simulink model "Projet_Final"  (R2024a)
settings: Solver=FixedStepAuto  StartTime=0.0  StopTime=6  FixedStep=Ts  RelTol=1e-3
values from neighbouring files (symbols this model uses):
  A1 = 0.548    [Parameters.m]
  A2 = 116    [Parameters.m]
  A3 = 0.4    [Parameters.m]
  A4 = 5    [Parameters.m]
  A5 = -21    [Parameters.m]
  A6 = 0.0068    [Parameters.m]
  C_Bat = 1e-3    (= 0.001)    [Parameters.m]    (also in Params_Battery_converter.m)
  C_dc = 4.5e-3    (= 0.0045)    [Parameters.m]
  f = 50    [Parameters.m]
  F = 0.0004924    [Parameters.m]
  G = 6.24    [Parameters.m]
  J = J_PMSG    (= 0.2227)    [Parameters.m]
  J_PMSG = 0.2227    [Parameters.m]
  ki_Ibat = 550    [Parameters.m]    (also in Params_Battery_converter.m)
  ki_id_grid = 225    [Parameters.m]
  ki_iq_grid = ki_id_grid    (= 225)    [Parameters.m]
  ki_isd = 13800    [Parameters.m]
  ki_omega = 0.6873    [Parameters.m]
  ki_PLL = 3200    [Parameters.m]
  ki_Q = 0.05    [Parameters.m]
  ki_vdc = C_dc * W_vdc^2    (= 28.8)    [Parameters.m]
  kp_Ibat = 6.28    [Parameters.m]    (also in Params_Battery_converter.m)
  kp_id_grid = 4.5    [Parameters.m]
  kp_iq_grid = kp_id_grid    (= 4.5)    [Parameters.m]
  kp_isd = 2.75    [Parameters.m]
  kp_omega = 3.108    [Parameters.m]
  kp_PLL = 180    [Parameters.m]
  kp_Q = 0.0005    [Parameters.m]
  kp_vdc = 2 * C_dc * W_vdc    (= 0.72)    [Parameters.m]
  Kt = 1.5 * p * Phi_r    (= 0.7164)    [Parameters.m]
  L_Bat = 2e-3    (= 0.002)    [Parameters.m]    (also in Params_Battery_converter.m)
  Lf = 8e-3    (= 0.008)    [Parameters.m]
  Ls = 0.000395    [Parameters.m]
  p = 4    [Parameters.m]
  Phi_r = 0.1194    [Parameters.m]
  R = 3.96    [Parameters.m]
  Rf = 0.01    [Parameters.m]
  rho = 1.225    [Parameters.m]
  Rs = 0.0485    [Parameters.m]
  S = pi*R^2    (= 49.2651993565)    [Parameters.m]
  Ts = 1e-6    (= 1e-06)    [Parameters.m]
  Vdc_ref = 700    [Parameters.m]    (also in Params_Battery_converter.m)
undefined symbols (not defined in the file or in its folder): Ion, Lithium
libraries: spsSeriesRLCBranchLib x19, slpidlib x11, spsMeanLib x6, spsThreePhaseVIMeasurementLib x6, spsThreePhaseBreakerLib x6, spsIdealSwitchLib x4, spsThreePhaseParallelRLCLoadLib x4, spsCurrentMeasurementLib x3, eeTransforms x3, spsPWMGenerator2LevelLib x3, spsVoltageMeasurementLib x3, spsUniversalBridgeLib x2
(part 3 of 3)

== system Projet_Final/Voltage Source Inverter (VSI)/GSC/boucle PLL, Calcul de PQ, Iabc to Idq grid ==
  note: P,Q Grid
  Enable_Sync : Inport
  Vabc : Inport  Port=2
  Iabc : Inport  Port=3
  Boucle PLL : Subsystem
  Demux2 : Demux  Outputs=3
      settings: DisplayOption=none
  Display : Display
      settings: Format=bank
  Display1 : Display
      settings: Format=bank
  Mean : spsMeanLib/Mean  Freq=50  Vinit=0  Ts=0
  Mean1 : spsMeanLib/Mean  Freq=50  Vinit=0  Ts=0
  Park Transform : eeTransforms/Park Transform  AxisAlignment=Q-axis  PowerInvariant=off
      settings: LibrarySourceBlock=|
      | ee_sl_lib/Mathematical
      | Transforms/Park Transform
  "Power (3ph, Instantaneous)" : spsPower3phInstantaneousLib/Power (3ph, Instantaneous)
  Product : Product
  Scope4 : Scope  NumInputPorts=2
  b1 : Terminator
  theta_grid : Scope
  id : Outport
  iq : Outport  Port=2
  theta_e : Outport  Port=3
  P : Outport  Port=4
  Q : Outport  Port=5
  wires:
  Boucle PLL/1(teta) -> theta_grid/1, theta_e/1, Park Transform/2
  Demux2/3 -> b1/1
  Park Transform/1 -> Demux2/1
  Iabc/1 -> Park Transform/1, "Power (3ph, Instantaneous)"/2
  Product/1 -> "Power (3ph, Instantaneous)"/1, Boucle PLL/1(Vabc)
  Mean/1 -> P/1, Scope4/1, Display/1
  Mean1/1 -> Q/1, Display1/1, Scope4/2
  "Power (3ph, Instantaneous)"/2 -> Mean1/1
  "Power (3ph, Instantaneous)"/1 -> Mean/1
  Demux2/2 -> iq/1
  Demux2/1 -> id/1
  Vabc/1 -> Product/2
  Enable_Sync/1 -> Product/1

== system Projet_Final/Wind Generation 20 kw/Wind Turbine/Power Coefficient Model Cp(λ, β) ==
  λ : Inport
  β : Inport  Port=2
  " Cp(λ,β)" : Fcn  Expr=A1 * ( ((A2 * u(2)) - (A3 * u(1)) - A4) * exp(A5 * u(2)) + (A6 * u(3)) )
  1/λi : Fcn  Expr=(1 / (u(2) + (0.08 * u(1)))) - (0.035 / ((u(1)^3) + 1))
  Mux : Mux  Inputs=2
  Mux1 : Mux  Inputs=3
  Cp : Outport
  wires:
  Mux1/1 -> " Cp(λ,β)"/1
  Mux/1 -> 1/λi/1
  λ/1 -> Mux/2, Mux1/3
  β/1 -> Mux/1, Mux1/1
  1/λi/1 -> Mux1/2
  " Cp(λ,β)"/1 -> Cp/1

== system Projet_Final/Wind Generation 20 kw/Wind Turbine/Subsystem ==
  Clock{,2..4} (4 alike) : Clock
  Escalier : MATLAB Function  TreatAsAtomicUnit=on
  MATLAB Function1 : MATLAB Function  TreatAsAtomicUnit=on  SystemSampleTime=0.001
  MATLAB Function3 : MATLAB Function  TreatAsAtomicUnit=on  SystemSampleTime=0.001
  MATLAB Function4 : MATLAB Function  TreatAsAtomicUnit=on  SystemSampleTime=0.001
  Nominal : Constant  Value=12
  Scope{1,7..9} (4 alike) : Scope
  V_wind : Outport
  wires:
  Clock2/1 -> MATLAB Function1/1(t)
  Clock4/1 -> MATLAB Function4/1(t)
  Escalier/1(signal) -> Scope9/1
  Clock/1 -> Escalier/1(t)
  MATLAB Function1/1(V_wind) -> Scope7/1
  MATLAB Function4/1(V_wind) -> Scope8/1
  Clock3/1 -> MATLAB Function3/1(t)
  Nominal/1 -> V_wind/1
  MATLAB Function3/1(V_wind) -> Scope1/1

== system Projet_Final/Active Rectifier/MSC/d-axis current controller with cross-coupling compensation/Decoupling Feedforward Terms ==
  note: Vd_ref = Vd_PI - (ω_e × Ls × isq)
  vd : Inport
  Iq : Inport  Port=2
  Wm : Inport  Port=3
  Product3 : Product  SaturateOnIntegerOverflow=on  OutDataTypeStr=Inherit: Same as first input
  Sum2 : Sum  Inputs=+-  SaturateOnIntegerOverflow=on
  u2 : Gain  Gain=Ls*p  SaturateOnIntegerOverflow=on  OutDataTypeStr=Inherit: Same as input  ParamDataTypeStr=Inherit: Same as input
  Vdref : Outport
  wires:
  Sum2/1 -> Vdref/1
  Wm/1 -> Product3/2
  Iq/1 -> Product3/1
  Product3/1 -> u2/1
  vd/1 -> Sum2/1
  u2/1 -> Sum2/2

== system Projet_Final/Active Rectifier/MSC/q-axis Current Controller with Cross-Coupling Compensation /DécouplaDecoupling Feedforward Termsge ==
  note: Vq_ref = Vq_PI + (ω_e × Ls × isd) + (ω_e × Φ_r)
  vq : Inport
  Id : Inport  Port=2
  Wm : Inport  Port=3
  Product3 : Product  SaturateOnIntegerOverflow=on  OutDataTypeStr=Inherit: Same as first input
  Sum2 : Sum  Inputs=+++  SaturateOnIntegerOverflow=on
  u1 : Gain  Gain=p*Phi_r  SaturateOnIntegerOverflow=on  OutDataTypeStr=Inherit: Same as input  ParamDataTypeStr=Inherit: Same as input
  u2 : Gain  Gain=p*Ls  SaturateOnIntegerOverflow=on  OutDataTypeStr=Inherit: Same as input  ParamDataTypeStr=Inherit: Same as input
  Vqref : Outport
  wires:
  vq/1 -> Sum2/1
  Product3/1 -> u2/1
  Id/1 -> Product3/1
  Wm/1 -> u1/1, Product3/2
  Sum2/1 -> Vqref/1
  u2/1 -> Sum2/2
  u1/1 -> Sum2/3

== system Projet_Final/Voltage Source Inverter (VSI)/GSC/Boucle id_grid // Tension Vdc/Découplage ==
  Vd : Inport
  iq_grid : Inport  Port=2
  Vd_grid : Inport  Port=3
  Gain : Gain  Gain=-2*pi*f*Lf
  Scope : Scope
  Sum : Sum  Inputs=+++
  Vd_ref : Outport
  wires:
  iq_grid/1 -> Gain/1
  Vd/1 -> Sum/2
  Gain/1 -> Sum/3
  Sum/1 -> Scope/1, Vd_ref/1
  Vd_grid/1 -> Sum/1

== system Projet_Final/Voltage Source Inverter (VSI)/GSC/Boucle iq_grid // Facteur de puissance/Subsystem ==
  Vq : Inport
  id_grid : Inport  Port=2
  Vq_grid : Inport  Port=3
  Gain : Gain  Gain=2*pi*f*Lf
  Scope : Scope
  Sum : Sum  Inputs=+++
  Vq_ref : Outport
  wires:
  id_grid/1 -> Gain/1
  Sum/1 -> Scope/1, Vq_ref/1
  Vq_grid/1 -> Sum/1
  Vq/1 -> Sum/2
  Gain/1 -> Sum/3

== system Projet_Final/Voltage Source Inverter (VSI)/GSC/boucle PLL, Calcul de PQ, Iabc to Idq grid/Boucle PLL ==
  Vabc : Inport
  Constant1 : Constant  Value=0
  Constant2 : Constant  Value=2*pi*50
  Demux : Demux  Outputs=3
  Integrator2 : Integrator
  Mux : Mux  Inputs=2
  PID Controller : slpidlib/PID Controller  Controller=PID  Form=Parallel  TimeDomain=Continuous-time  UseExternalTs=off  SampleTime=-1  IntegratorMethod=Forward Euler  FilterMethod=Forward Euler  ControllerParametersSource=internal  P=kp_PLL  I=ki_PLL  UseKiTs=off  D=0  UseExternalDerivativeSource=off  N=100  UseFilter=on  TunerSelectOption=Transfer Function Based (PID Tuner App)  InitialConditionSource=internal  InitialConditionForIntegrator=0  InitialConditionForFilter=0  DifferentiatorICPrevScaledInput=0  ExternalReset=none  TrackingMode=off  Kt=1  LimitOutput=off  SatLimitsSource=internal  UpperSaturationLimit=inf  LowerSaturationLimit=-inf  LinearizeAsGain=on  AntiWindupMode=none  Kb=1  LimitIntegrator=off  UpperIntegratorSaturationLimit=inf  LowerIntegratorSaturationLimit=-inf  POutMin=[]  POutMax=[]  IOutMin=[]  IOutMax=[]  DOutMin=[]  DOutMax=[]  NOutMin=[]  NOutMax=[]  SumOutMin=[]  SumOutMax=[]  SaturationOutMin=[]  SaturationOutMax=[]  PParamMin=[]  PParamMax=[]  IParamMin=[]  IParamMax=[]  DParamMin=[]  DParamMax=[]  NParamMin=[]  NParamMax=[]  KbParamMin=[]  KbParamMax=[]  KtParamMin=[]  KtParamMax=[]  KbOutMin=[]  KbOutMax=[]  KtOutMin=[]  KtOutMax=[]  IntegratorOutMin=[]  IntegratorOutMax=[]  FilterOutMin=[]  FilterOutMax=[]  SumI1OutMin=[]  SumI1OutMax=[]  SumI2OutMin=[]  SumI2OutMax=[]  SumI3OutMin=[]  SumI3OutMax=[]  SumI4OutMin=[]  SumI4OutMax=[]  SumDOutMin=[]  SumDOutMax=[]  DifferentiatorOutMin=[]  DifferentiatorOutMax=[]  FilterDiffOutCoefMin=[]  FilterDiffOutCoefMax=[]  ReciprocalOutMin=[]  ReciprocalOutMax=[]  SumDenOutMin=[]  SumDenOutMax=[]  SumNumOutMin=[]  SumNumOutMax=[]  DivideOutMin=[]  DivideOutMax=[]  UdiffTsProdOutMin=[]  UdiffTsProdOutMax=[]  NTsProdOutMin=[]  NTsProdOutMax=[]  UintegralTsProdOutMin=[]  UintegralTsProdOutMax=[]  UngainTsProdOutMin=[]  UngainTsProdOutMax=[]  ClampingZeroOutDataTypeStr=Inherit: Inherit via back propagation  ClampingZeroOutMin=[]  ClampingZeroOutMax=[]  FilterDenConstantOutDataTypeStr=Inherit: Inherit via back propagation  FilterDenConstantOutMin=[]  FilterDenConstantOutMax=[]  PCopyOutDataTypeStr=Inherit: Inherit via back propagation  PCopyOutMin=[]  PCopyOutMax=[]  NCopyOutDataTypeStr=Inherit: Inherit via back propagation  NCopyOutMin=[]  NCopyOutMax=[]  IntegratorContinuousStateAttributes=''  IntegratorStateMustResolveToSignalObject=off  IntegratorRTWStateStorageClass=Auto  FilterContinuousStateAttributes=''  FilterStateMustResolveToSignalObject=off  FilterRTWStateStorageClass=Auto  ParallelPVariant=InternalParameters  IdealPVariant=Disabled  IVariant=InternalParameters  DVariant=InternalParameters  IntegratorVariant=Continuous  SatVariant=Disabled  AWVariant=Passthrough  PCopyVariant=Disabled  TRVariant=Disabled  FdbkBlocksVariant=Forward  IdealPFdbkVariant=Disabled  SatFdbkVariant=Disabled  DerivativeFilterVariant=ContFilter  NVariant=InternalParameters  NCopyVariant=Disabled  FilterICVariant=InternalICsFilter  IntegratorICVariant=InternalICs  ExternalResetVariant=Disabled  TRSumVariant=Passthrough  SumFdbkVariant=Disabled  SumVariant=Sum_PID  TsampFilterVariant=InternalTs  TsampNgainVariant=Passthrough  TsampIntegralVariant=Disabled_SignalSpec  ExternalSaturationOutDataTypeStr=Inherit: Same as second input  DerivativeSourceVariant=ErrorSignal
  Sum1 : Sum  SaturateOnIntegerOverflow=on
  Sum3 : Sum  Inputs=+-  SaturateOnIntegerOverflow=on
  Trigonometric Function : Trigonometry
  Trigonometric Function1 : Trigonometry  Operator=cos
  abc_to_dq0 Transformation1 : powerlib_extras/Measurements/abc_to_dq0 Transformation
  b1 : Terminator
  teta : Outport
  tag scope: Vd_grid=global, Vq_grid=global
  wires:
  Demux/1 -> [Vd_grid]
  Mux/1 -> abc_to_dq0 Transformation1/2
  Trigonometric Function1/1 -> Mux/2
  Trigonometric Function/1 -> Mux/1
  abc_to_dq0 Transformation1/1 -> Demux/1
  Integrator2/1 -> Trigonometric Function/1, Trigonometric Function1/1, teta/1
  Sum3/1 -> PID Controller/1
  PID Controller/1 -> Sum1/2
  Constant2/1 -> Sum1/1
  Sum1/1 -> Integrator2/1
  Constant1/1 -> Sum3/1
  Vabc/1 -> abc_to_dq0 Transformation1/1
  Demux/2 -> Sum3/2, [Vq_grid]
  Demux/3 -> b1/1

== matlab function Projet_Final/Bidirectional DC–DC Converter/MATLAB Function ==
  data: SOC input; Bat_Enable output
function Bat_Enable = Battery_Protection(SOC)

SOC_min = 20;
SOC_max = 90;

if SOC <= SOC_min
    Bat_Enable = 0;
elseif SOC >= SOC_max
    Bat_Enable = 0;
else
    Bat_Enable = 1;
end

end

== matlab function Projet_Final/Wind Generation 20 kw/Wind Turbine/Subsystem/Escalier ==
  data: t input; signal output
function signal = generate_step_signal(t)
    % Génère un signal qui varie par paliers constants sur 20 secondes
    % Input : vecteur temps t (en secondes)
    % Output : signal avec des valeurs constantes par segment
    
    signal = zeros(size(t));  % Initialisation du signal
    
    % Définition des intervalles de temps (en secondes) et des valeurs constantes
    segments = [
        0,  4,  12;   % De 0 à 4 sec : valeur = 2.5
        4,  8,  16;   % De 4 à 8 sec : valeur = 1.0
        8,  12, 8;   % De 8 à 12 sec : valeur = 4.0
        12, 16, 14;   % De 12 à 16 sec : valeur = 3.2
        16, 20, 18;   % De 16 à 20 sec : valeur = 0.5
    ];
    
    % Génération du signal par morceaux
    for i = 1:size(segments, 1)
        start_time = segments(i, 1);
        end_time = segments(i, 2);
        value = segments(i, 3);
        
        mask = (t >= start_time) & (t < end_time);
        signal(mask) = value;
    end
    
    % Gestion de la dernière valeur (t = 20)
    signal(t == 20) = segments(end, 3);
end

== matlab function Projet_Final/Wind Generation 20 kw/PMSG/MATLAB Function ==
  data: t input; V_vent input; T_startup output; Omega_ref_init output; Starter_Off output; Omega_mes input; P_cible input; Omega_cible input
function [T_startup, Omega_ref_init, Starter_Off] = Demarreur(t, V_vent, Omega_mes, P_cible, Omega_cible)

    persistent startup_done
    
    if isempty(startup_done)
        startup_done = 0;
    end
      

    T_25kW = P_cible / Omega_cible; 
    
    T_startup = T_25kW;
    Omega_ref_init = Omega_cible;

    
    Seuil_Vitesse_Haute = Omega_cible*0.99;


    if (Omega_mes >= Seuil_Vitesse_Haute) && (V_vent > 5) && (t >= 0.6)
        startup_done = 1; 
        T_startup = 0;
    end
    Starter_Off = startup_done;
end

== matlab function Projet_Final/Wind Generation 20 kw/Wind Turbine/Subsystem/MATLAB Function3 ==
  data: t input; V_wind output
function V_wind = Wind_Profile1(t)
%#codegen
% Profil de vent à rampes avec valeur moyenne = 12 m/s

time_points  = [0.0, 2.0, 5.0, 7.5, 10.0, 15.0, 20.0];
speed_points = [10.3, 11.87, 8, 9, 13, 9, 10];

if t < time_points(1)
    V_wind = speed_points(1);
    return;
end

if t > time_points(end)
    V_wind = speed_points(end);
    return;
end

V_wind = interp1(time_points, speed_points, t, 'linear');

end

== matlab function Projet_Final/Wind Generation 20 kw/Wind Turbine/Subsystem/MATLAB Function1 ==
  data: t input; V_wind output
function V_wind = Wind_Profile2(t)
    % Fonction de profil de vent avec contraintes spécifiques
    % Moyenne = 12, Max = 20, Min = 5
    
    % Points temporels
    time_points = [0.0, 2.0, 5.0, 7.5, 10.0, 15.0, 20.0];
    
    % Nouvelles valeurs ajustées pour respecter les contraintes
    % Calculées pour avoir: moyenne=12, min=5, max=20
    speed_points = [8.5, 12.5, 20, 16.0, 10.5, 5.0, 10.5];
    
    % Gestion des limites temporelles (nécessaire pour Code Generation)
    if t <= time_points(1)
        V_wind = speed_points(1);
    elseif t >= time_points(end)
        V_wind = speed_points(end);
    else
        % Interpolation linéaire
        % Pour la génération de code, utiliser une implémentation manuelle
        V_wind = linear_interp(time_points, speed_points, t);
    end
end

function y = linear_interp(x_vec, y_vec, x)
    % Interpolation linéaire manuelle pour la génération de code
    n = length(x_vec);
    
    % Trouver l'intervalle
    for i = 1:n-1
        if x >= x_vec(i) && x <= x_vec(i+1)
            % Interpolation linéaire
            dx = x_vec(i+1) - x_vec(i);
            if abs(dx) < eps
                y = y_vec(i);
            else
                t = (x - x_vec(i)) / dx;
                y = y_vec(i) + t * (y_vec(i+1) - y_vec(i));
            end
            return;
        end
    end
    
    % Si on arrive ici (ne devrait pas arriver avec les vérifications ci-dessus)
    y = y_vec(end);
end

== matlab function Projet_Final/Active Rectifier/      /MATLAB Function2 ==
  data: P_mes input; Omega_ref output; P_betz input; Omega_Start input; Activation input
function Omega_ref = MPPT_Adaptive_PO (P_mes, P_betz,Omega_Start, Activation)
%#codegen
persistent P_prev Omega_ref_prev direction initialized counter;

% --- PARAMÈTRES ---
Omega_min = Omega_Start;
Omega_max = 350;
Eff_est   = 1;

% --- Initialisation ---
if isempty(initialized)
    P_prev = 0;
    Omega_ref_prev = Omega_Start; 
    direction = 1; 
    counter = 0;
    initialized = true;
end

% --- 1. GESTION DU DÉMARRAGE ---
if Activation == 0
    Omega_ref = Omega_Start;
    Omega_ref_prev = Omega_Start; 
    P_prev = P_mes;
    return;
end

% --- 2. TEMPORISATION ---
if counter < 50
    counter = counter + 1;
    Omega_ref = Omega_ref_prev;
    return;
end
counter = 0;

% --- 3. CALCUL DU PAS VARIABLE (MODIFIÉ POUR RAPIDITÉ) ---
P_target = P_betz * Eff_est;
Erreur_P = abs(P_target - P_mes); 

if Erreur_P > 1500
    % Grand écart : Réaction très forte
    Step_Size = 8; 
elseif Erreur_P > 500
    % Écart moyen (Cas t=2s) : Vitesse triplée (passé de 1 à 3)
    Step_Size = 3;  
elseif Erreur_P < 10
    % Zone morte (Stabilisation)
    Step_Size = 0; 
else
    % Ajustement fin
    Step_Size = 0.4; 
end

% --- 4. LOGIQUE P&O STANDARD ---
delta_P = P_mes - P_prev;

% Inversion de direction si la puissance chute
if delta_P < -50
    direction = -direction; 
end

% --- 5. CALCUL FINAL ---
Omega_ref = Omega_ref_prev + (direction * Step_Size);
Omega_ref = max(Omega_min, min(Omega_ref, Omega_max));

% Mises à jour
P_prev = P_mes;
Omega_ref_prev = Omega_ref;

end

== matlab function Projet_Final/Active Rectifier/      /MATLAB Function3 ==
  data: V_vent input; P_aero_ref output
function P_aero_ref = Estimateur_Paero(V_vent)
%#codegen
% ESTIMATEUR_PAERO
% Calcule la puissance aérodynamique maximale théorique (P_aero)
% basée sur le Cp_max identifié.

% --- Paramètres Physiques ---
R = 3.96;             % Rayon pale (m)
rho = 1.225;          % Densité air (kg/m^3)
Cp_max = 0.48;        % Coefficient de puissance max (donnée)

% --- Calcul du Gain Optimal (K_opt) ---
% S = Surface balayée (m^2)
S = pi * R^2;

% K_opt = 0.5 * rho * S * Cp_max
% Avec les valeurs : 0.5 * 1.225 * 49.265 * 0.48 ≈ 14.48
K_opt = 0.5 * rho * S * Cp_max;

% --- Calcul de la Puissance Aérodynamique ---
% P = K_opt * V^3
P_aero_ref = K_opt * (V_vent^3);

end

== matlab function Projet_Final/Wind Generation 20 kw/Wind Turbine/Subsystem/MATLAB Function4 ==
  data: t input; V_wind output
function V_wind = Wind_Profile3(t)
%#codegen
% Profil de vent à rampes avec valeur moyenne = 12 m/s

time_points  = [2, 4, 6, 8, 10, 12, 14, 16, 18, 20];
speed_points = [5, 8, 12, 10, 13, 7, 10, 16, 15, 12 ];

if t < time_points(1)
    V_wind = speed_points(1);
    return;
end

if t > time_points(end)
    V_wind = speed_points(end);
    return;
end

V_wind = interp1(time_points, speed_points, t, 'linear');

end
